simulink model "R2_integrator"  (R2014b)
settings: Solver=ode3  SolverMode=SingleTasking  StartTime=0.0  StopTime=Tsim  FixedStep=Ts  RelTol=1e-3
InitFcn:
  | configIntegrator
settings Model: CovMetricSettings=dwe  CovHtmlReporting=off  covSaveCumulativeToWorkspaceVar=off  CovSaveSingleToWorkspaceVar=off  CovExternalEMLEnable=on  CovSFcnEnable=on  Creator=mnade  LastModifiedBy=nina
settings DataIOCC: LimitDataPoints=off  SaveFormat=StructureWithTime
settings DebuggingCC: SolverPrmCheckMsg=none  FrameProcessingCompatibilityMsg=error  SFUnexpectedBacktrackingDiag=error  SFNoUnconditionalDefaultTransitionDiag=error
settings HardwareCC: ProdBitPerPointer=64  ProdLargestAtomicFloat=Float  ProdIntDivRoundTo=Zero  ProdEndianess=LittleEndian  ProdHWDeviceType=Specified
settings ModelReferenceCC: PropagateSignalLabelsOutOfModel=on
settings GRTTargetCC: TargetLangStandard=C99 (ISO)  GeneratePreprocessorConditionals=Use local settings

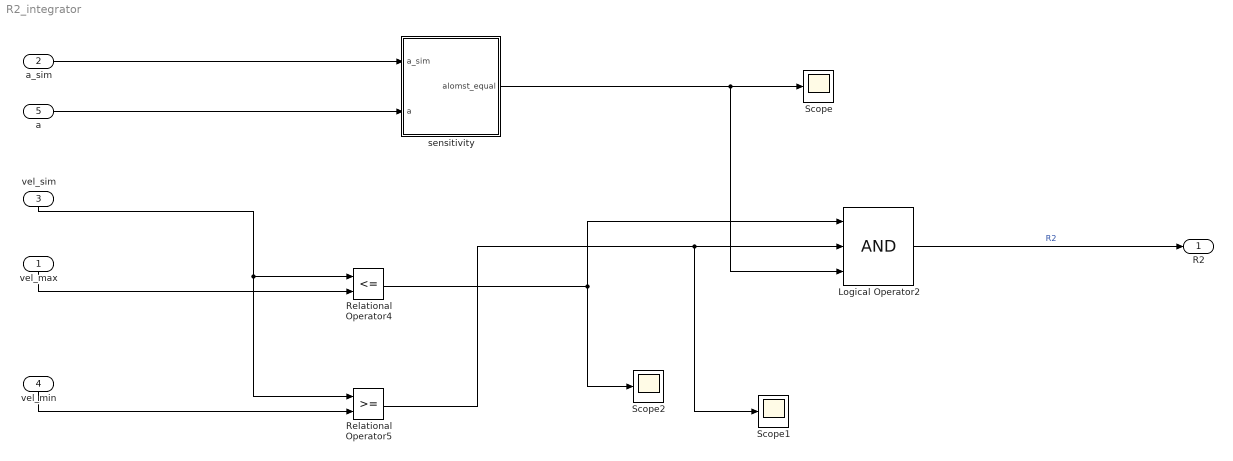
== system R2_integrator ==
  vel_max : Inport
  a_sim : Inport  Port=2
  vel_sim : Inport  Port=3
  vel_min : Inport  Port=4
  a : Inport  Port=5
  Logical Operator2 : Logic  Inputs=3  AllPortsSameDT=off  OutDataTypeStr=boolean
  Relational Operator4 : RelationalOperator  Operator=<=  OutDataTypeStr=boolean
  Relational Operator5 : RelationalOperator  OutDataTypeStr=boolean
  Scope : Scope
  Scope1 : Scope
  Scope2 : Scope
      settings: SaveName=ScopeData2
  sensitivity : Subsystem
  R2 : Outport
  wires:
  Logical Operator2/1 -> R2/1  "R2"
  vel_max/1 -> Relational Operator4/2
  vel_min/1 -> Relational Operator5/2
  Relational Operator4/1 -> Logical Operator2/1, Scope2/1
  Relational Operator5/1 -> Scope1/1, Logical Operator2/2
  vel_sim/1 -> Relational Operator5/1, Relational Operator4/1
  sensitivity/1(alomst_equal) -> Scope/1, Logical Operator2/3
  a_sim/1 -> sensitivity/1(a_sim)
  a/1 -> sensitivity/2(a)

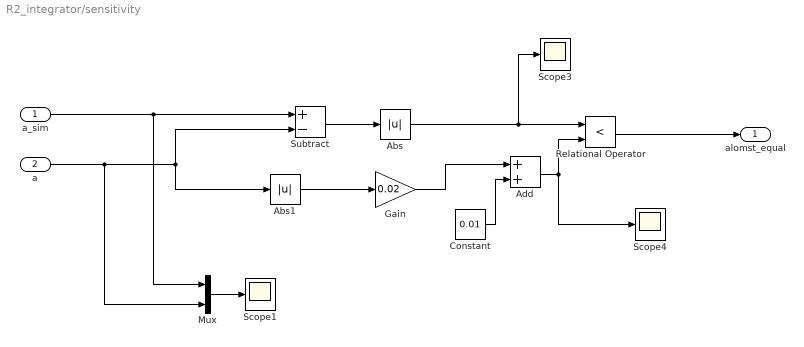
== system R2_integrator/sensitivity ==
  a_sim : Inport
  a : Inport  Port=2
  Abs : Abs
  Abs1 : Abs
  Add : Sum
  Constant : Constant  Value=0.01
  Gain : Gain  Gain=0.02
  Mux : Mux  Inputs=2
  Relational Operator : RelationalOperator  Operator=<  OutDataTypeStr=boolean
  Scope1 : Scope
      settings: SaveName=ScopeData5
  Scope3 : Scope
      settings: SaveName=ScopeData3
  Scope4 : Scope
      settings: SaveName=ScopeData4
  Subtract : Sum  Inputs=+-
  alomst_equal : Outport
  wires:
  a/1 -> Mux/2, Subtract/2, Abs1/1
  Gain/1 -> Add/1
  Abs1/1 -> Gain/1
  Abs/1 -> Scope3/1, Relational Operator/1
  Add/1 -> Scope4/1, Relational Operator/2
  Subtract/1 -> Abs/1
  Constant/1 -> Add/2
  a_sim/1 -> Mux/1, Subtract/1
  Relational Operator/1 -> alomst_equal/1
  Mux/1 -> Scope1/1
